simulink model "SiC_Mosfet_model"  (R2019a)
settings: Solver=VariableStepAuto  StartTime=0.0  StopTime=10.0  RelTol=1e-3
libraries: nesl_utility x10, ee_lib x7, fl_lib x3
settings Model: Creator=karth  LastModifiedBy=karth

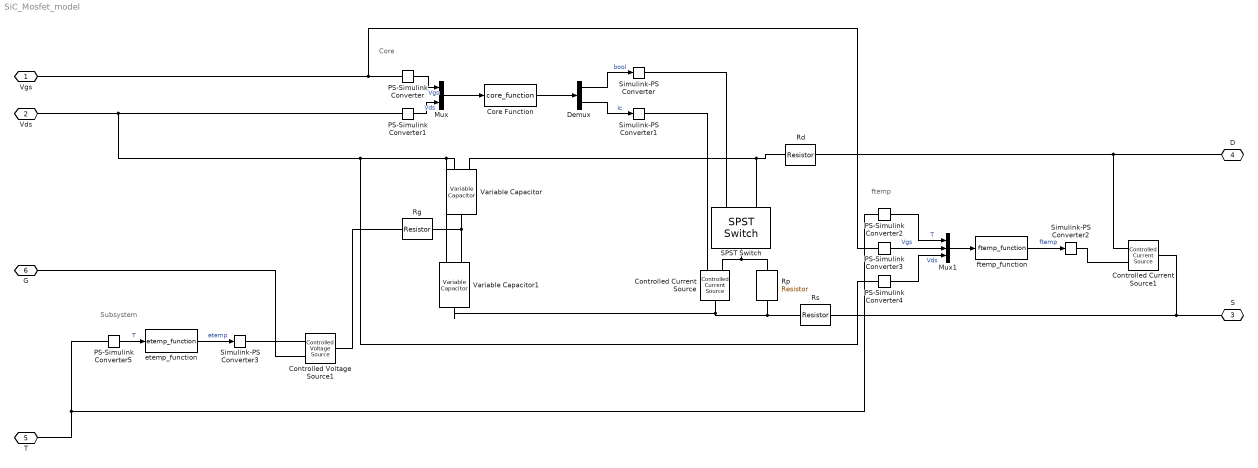
== system SiC_Mosfet_model ==
  note: Subsystem
  note: ftemp
  note: Core
  Controlled Current Source : fl_lib/Electrical/Electrical Sources/Controlled Current Source
  Controlled Current Source1 : fl_lib/Electrical/Electrical Sources/Controlled Current Source
  Controlled Voltage Source1 : fl_lib/Electrical/Electrical Sources/Controlled Voltage Source
  Core Function : MATLABFcn  MATLABFcn=core_function
  Demux : Demux  Outputs=2
  Mux : Mux  Inputs=2
  Mux1 : Mux  Inputs=3
  PS-Simulink Converter{,1..5} (6 alike) : nesl_utility/PS-Simulink Converter  PhysicalDomain=network_engine_domain  SubClassName=ps_output  LeftPortType=input  RightPortType=output  PseudoPeriodic=off  Frequencies=[]  Unit=1  AffineConversion=off
  Rd : ee_lib/Passive/Resistor  R=1 Ohm  R_tol=5  enable_R_tol=0  tol_distribution=1  nSigma=4  enable_operating_limits=0  operating_limit_action=2  max_working_voltage=100 V  power_rating=1 W  enable_faults=0  fault_action=1  R_faulted=inf Ohm  enable_temporal_fault=0  t_fault=1 s  enable_behavioral_fault=0  max_permissible_current=1 A  t_fail_on_current=1 s  noise_mode=0  sample_time=1e-3 s  repeatability=1  auto_seed=2715962282  user_seed=0  Tdevice=25 degC  alpha=3.93e-3 1/K  Tmeas=25 degC  thermal_mass=100 J/K  power_derating_T1=70 degC  power_derating_T2=155 degC  operating_temperature_range_vec=[-50, 150] degC  temperature_specify=off  temperature_priority=High  temperature=298.15 K  temperature_nominal_specify=off  temperature_nominal_unit=K  temperature_nominal_value=1
      settings: SourceProductName=Simscape Electrical
  Rg : ee_lib/Passive/Resistor  R=1 Ohm  R_tol=5  enable_R_tol=0  tol_distribution=1  nSigma=4  enable_operating_limits=0  operating_limit_action=2  max_working_voltage=100 V  power_rating=1 W  enable_faults=0  fault_action=1  R_faulted=inf Ohm  enable_temporal_fault=0  t_fault=1 s  enable_behavioral_fault=0  max_permissible_current=1 A  t_fail_on_current=1 s  noise_mode=0  sample_time=1e-3 s  repeatability=1  auto_seed=418932850  user_seed=0  Tdevice=25 degC  alpha=3.93e-3 1/K  Tmeas=25 degC  thermal_mass=100 J/K  power_derating_T1=70 degC  power_derating_T2=155 degC  operating_temperature_range_vec=[-50, 150] degC  temperature_specify=off  temperature_priority=High  temperature=298.15 K  temperature_nominal_specify=off  temperature_nominal_unit=K  temperature_nominal_value=1
      settings: SourceProductName=Simscape Electrical
  Rp : ee_lib/Passive/Resistor  R=1 Ohm  R_tol=5  enable_R_tol=0  tol_distribution=1  nSigma=4  enable_operating_limits=0  operating_limit_action=2  max_working_voltage=100 V  power_rating=1 W  enable_faults=0  fault_action=1  R_faulted=inf Ohm  enable_temporal_fault=0  t_fault=1 s  enable_behavioral_fault=0  max_permissible_current=1 A  t_fail_on_current=1 s  noise_mode=0  sample_time=1e-3 s  repeatability=1  auto_seed=1196140742  user_seed=0  Tdevice=25 degC  alpha=3.93e-3 1/K  Tmeas=25 degC  thermal_mass=100 J/K  power_derating_T1=70 degC  power_derating_T2=155 degC  operating_temperature_range_vec=[-50, 150] degC  temperature_specify=off  temperature_priority=High  temperature=298.15 K  temperature_nominal_specify=off  temperature_nominal_unit=K  temperature_nominal_value=1
      settings: SourceProductName=Simscape Electrical
  Rs : ee_lib/Passive/Resistor  R=1 Ohm  R_tol=5  enable_R_tol=0  tol_distribution=1  nSigma=4  enable_operating_limits=0  operating_limit_action=2  max_working_voltage=100 V  power_rating=1 W  enable_faults=0  fault_action=1  R_faulted=inf Ohm  enable_temporal_fault=0  t_fault=1 s  enable_behavioral_fault=0  max_permissible_current=1 A  t_fail_on_current=1 s  noise_mode=0  sample_time=1e-3 s  repeatability=1  auto_seed=2348838240  user_seed=0  Tdevice=25 degC  alpha=3.93e-3 1/K  Tmeas=25 degC  thermal_mass=100 J/K  power_derating_T1=70 degC  power_derating_T2=155 degC  operating_temperature_range_vec=[-50, 150] degC  temperature_specify=off  temperature_priority=High  temperature=298.15 K  temperature_nominal_specify=off  temperature_nominal_unit=K  temperature_nominal_value=1
      settings: SourceProductName=Simscape Electrical
  SPST Switch : ee_lib/Switches & Breakers/SPST Switch  R_closed=0.01 Ohm  G_open=1e-6 S  Threshold=0.5 V  Width=0 V  model_dynamics=0  t_on=1e-3 s  t_off=1e-3 s  initial_vT=0 V
      settings: SourceProductName=Simscape Electrical  SourceProductBaseCode=PS
  Simulink-PS Converter{,1..3} (4 alike) : nesl_utility/Simulink-PS Converter  PhysicalDomain=network_engine_domain  SubClassName=ps_input  LeftPortType=input  RightPortType=output  PseudoPeriodic=off  Frequencies=[]  NoiseDistribution=none  NoiseParameters=[]  Unit=1  AffineConversion=off  FilteringAndDerivatives=provide  SimscapeFilterOrder=1  InputFilterTimeConstant=0.001  UdotUserProvided=0
  Variable Capacitor : ee_lib/Passive/Variable Capacitor  prm=2  Cmin=1e-9 F  r=1e-6 Ohm  v0=0 V  q0=0 C
      settings: SourceProductName=Simscape Electrical  SourceProductBaseCode=PS
  Variable Capacitor1 : ee_lib/Passive/Variable Capacitor  prm=2  Cmin=1e-9 F  r=1e-6 Ohm  v0=0 V  q0=0 C
      settings: SourceProductName=Simscape Electrical  SourceProductBaseCode=PS
  etemp_function : MATLABFcn  MATLABFcn=etemp_function
  ftemp_function : MATLABFcn  MATLABFcn=ftemp_function
  Vgs : PMIOPort  Side=Left
  Vds : PMIOPort  Port=2  Side=Left
  S : PMIOPort  Port=3  Side=Left
  D : PMIOPort  Port=4  Side=Left
  T : PMIOPort  Port=5  Side=Left
  G : PMIOPort  Port=6  Side=Left
  wires:
  Demux/1 -> Simulink-PS Converter/1  "bool"
  PS-Simulink Converter/1 -> Mux/1  "Vgs"
  Core Function/1 -> Demux/1
  PS-Simulink Converter1/1 -> Mux/2  "Vds"
  Demux/2 -> Simulink-PS Converter1/1  "Ic"
  Mux/1 -> Core Function/1
  Mux1/1 -> ftemp_function/1
  PS-Simulink Converter3/1 -> Mux1/2  "Vgs"
  PS-Simulink Converter2/1 -> Mux1/1  "T"
  PS-Simulink Converter4/1 -> Mux1/3  "Vds"
  ftemp_function/1 -> Simulink-PS Converter2/1  "ftemp"
  PS-Simulink Converter5/1 -> etemp_function/1  "T"
  etemp_function/1 -> Simulink-PS Converter3/1  "etemp"
  connections:
  Rs/LConn1 -- Controlled Current Source1/LConn1 -- S/RConn1
  Rd/LConn1 -- Controlled Current Source1/RConn2 -- D/RConn1
  PS-Simulink Converter1/LConn1 -- Variable Capacitor1/LConn1 -- Variable Capacitor/LConn1 -- PS-Simulink Converter4/LConn1 -- Vds/RConn1
  PS-Simulink Converter/LConn1 -- Vgs/RConn1 -- PS-Simulink Converter3/LConn1
  Controlled Voltage Source1/LConn1 -- Rg/RConn1
  Simulink-PS Converter/RConn1 -- SPST Switch/LConn1
  Rg/LConn1 -- Variable Capacitor/RConn1 -- Variable Capacitor1/LConn2
  Simulink-PS Converter1/RConn1 -- Controlled Current Source/RConn1
  SPST Switch/RConn1 -- Rp/LConn1 -- Controlled Current Source/RConn2
  Variable Capacitor/LConn2 -- Rd/RConn1 -- SPST Switch/LConn2
  Rp/RConn1 -- Rs/RConn1 -- Variable Capacitor1/RConn1 -- Controlled Current Source/LConn1
  PS-Simulink Converter2/LConn1 -- T/RConn1 -- PS-Simulink Converter5/LConn1
  Simulink-PS Converter2/RConn1 -- Controlled Current Source1/RConn1
  Controlled Voltage Source1/RConn1 -- Simulink-PS Converter3/RConn1
  Controlled Voltage Source1/RConn2 -- G/RConn1
